simulink model "Model_vs_Real_control"  (R2019b)
settings: Solver=FixedStepAuto  StartTime=0.0  StopTime=10  FixedStep=1e-3  RelTol=1e-3
values from neighbouring files (symbols this model uses):
  N = 1/Tf    [HorizontalBeamControl.m]
  V_max = 10    [HorizontalBeamControl.m]
undefined symbols (not defined in the file or in its folder): Kd, Ki, Kp, Parameters, tf2_1, tf2_2
libraries: simulink x4
settings Model: Creator=Guido  LastModifiedBy=pietr

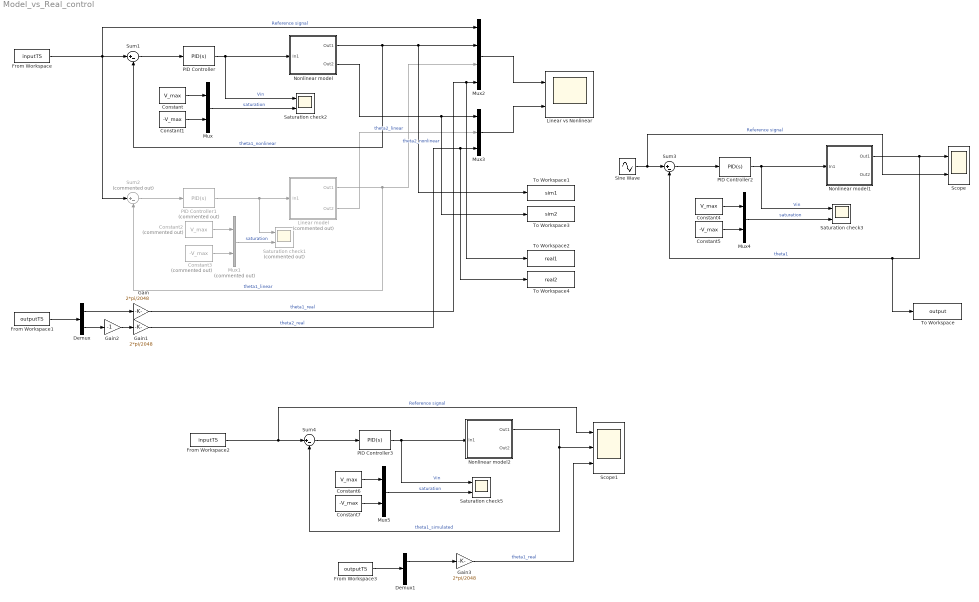
== system Model_vs_Real_control ==
  Constant : Constant  Value=V_max
  Constant1 : Constant  Value=-V_max
  Constant2 : Constant  Commented=on  Value=V_max
  Constant3 : Constant  Commented=on  Value=-V_max
  Constant4 : Constant  Value=V_max
  Constant5 : Constant  Value=-V_max
  Constant6 : Constant  Value=V_max
  Constant7 : Constant  Value=-V_max
  Demux : Demux  Outputs=2
  Demux1 : Demux  Outputs=2
  From Workspace : FromWorkspace  VariableName=inputTS  SampleTime=0
  From Workspace1 : FromWorkspace  VariableName=outputTS  SampleTime=0
  From Workspace2 : FromWorkspace  VariableName=inputTS  SampleTime=0
  From Workspace3 : FromWorkspace  VariableName=outputTS  SampleTime=0
  Gain : Gain  Gain=2*pi/2048
  Gain1 : Gain  Gain=2*pi/2048
  Gain2 : Gain  Gain=-1
  Gain3 : Gain  Gain=2*pi/2048
  Linear model : Subsystem  Commented=on
  Linear vs Nonlinear : Scope  NumInputPorts=2
  Mux : Mux  Inputs=2
  Mux1 : Mux  Commented=on  Inputs=2
  Mux2 : Mux
  Mux3 : Mux  Inputs=3
  Mux4 : Mux  Inputs=2
  Mux5 : Mux  Inputs=2
  Nonlinear model : Subsystem
  Nonlinear model1 : Subsystem
  Nonlinear model2 : Subsystem
  PID Controller : simulink/Continuous/PID Controller  Controller=PID  Form=Parallel  TimeDomain=Continuous-time  SampleTime=-1  IntegratorMethod=Forward Euler  FilterMethod=Forward Euler  ControllerParametersSource=internal  P=Kp  I=Ki  D=Kd  UseFilter=on  N=N  TunerSelectOption=Transfer Function Based (PID Tuner App)  InitialConditionSource=internal  InitialConditionForIntegrator=0  InitialConditionForFilter=0  DifferentiatorICPrevScaledInput=0  ExternalReset=none  TrackingMode=off  Kt=1  LimitOutput=on  UpperSaturationLimit=V_max  LowerSaturationLimit=-V_max  LinearizeAsGain=on  AntiWindupMode=back-calculation  Kb=1  POutMin=[]  POutMax=[]  IOutMin=[]  IOutMax=[]  DOutMin=[]  DOutMax=[]  NOutMin=[]  NOutMax=[]  SumOutMin=[]  SumOutMax=[]  SaturationOutMin=[]  SaturationOutMax=[]  PParamMin=[]  PParamMax=[]  IParamMin=[]  IParamMax=[]  DParamMin=[]  DParamMax=[]  NParamMin=[]  NParamMax=[]  KbParamMin=[]  KbParamMax=[]  KtParamMin=[]  KtParamMax=[]  KbOutMin=[]  KbOutMax=[]  KtOutMin=[]  KtOutMax=[]  IntegratorOutMin=[]  IntegratorOutMax=[]  FilterOutMin=[]  FilterOutMax=[]  SumI1OutMin=[]  SumI1OutMax=[]  SumI2OutMin=[]  SumI2OutMax=[]  SumI3OutMin=[]  SumI3OutMax=[]  SumI4OutMin=[]  SumI4OutMax=[]  SumDOutMin=[]  SumDOutMax=[]  DifferentiatorOutMin=[]  DifferentiatorOutMax=[]  FilterDiffOutCoefMin=[]  FilterDiffOutCoefMax=[]  ReciprocalOutMin=[]  ReciprocalOutMax=[]  SumDenOutMin=[]  SumDenOutMax=[]  SumNumOutMin=[]  SumNumOutMax=[]  DivideOutMin=[]  DivideOutMax=[]  IntegratorContinuousStateAttributes=''  IntegratorStateMustResolveToSignalObject=off  IntegratorRTWStateStorageClass=Auto  FilterContinuousStateAttributes=''  FilterStateMustResolveToSignalObject=off  FilterRTWStateStorageClass=Auto  ParallelPVariant=InternalParameters  IdealPVariant=Disabled  IVariant=InternalParameters  DVariant=InternalParameters  IntegratorVariant=Continuous  SatVariant=Enabled  AWVariant=BackCalculation  PCopyVariant=Disabled  TRVariant=Disabled  FdbkBlocksVariant=Forward  IdealPFdbkVariant=Disabled  SatFdbkVariant=Disabled  DerivativeFilterVariant=ContFilter  NVariant=InternalParameters  NCopyVariant=Disabled  FilterICVariant=InternalICsFilter  IntegratorICVariant=InternalICs  ExternalResetVariant=Disabled  TRSumVariant=Passthrough  SumFdbkVariant=Disabled  SumVariant=Sum_PID
  PID Controller1 : simulink/Continuous/PID Controller  Commented=on  Controller=PID  Form=Parallel  TimeDomain=Continuous-time  SampleTime=-1  IntegratorMethod=Forward Euler  FilterMethod=Forward Euler  ControllerParametersSource=internal  P=Kp  I=Ki  D=Kd  UseFilter=on  N=N  TunerSelectOption=Transfer Function Based (PID Tuner App)  InitialConditionSource=internal  InitialConditionForIntegrator=0  InitialConditionForFilter=0  DifferentiatorICPrevScaledInput=0  ExternalReset=none  TrackingMode=off  Kt=1  LimitOutput=on  UpperSaturationLimit=V_max  LowerSaturationLimit=-V_max  LinearizeAsGain=on  AntiWindupMode=back-calculation  Kb=1  POutMin=[]  POutMax=[]  IOutMin=[]  IOutMax=[]  DOutMin=[]  DOutMax=[]  NOutMin=[]  NOutMax=[]  SumOutMin=[]  SumOutMax=[]  SaturationOutMin=[]  SaturationOutMax=[]  PParamMin=[]  PParamMax=[]  IParamMin=[]  IParamMax=[]  DParamMin=[]  DParamMax=[]  NParamMin=[]  NParamMax=[]  KbParamMin=[]  KbParamMax=[]  KtParamMin=[]  KtParamMax=[]  KbOutMin=[]  KbOutMax=[]  KtOutMin=[]  KtOutMax=[]  IntegratorOutMin=[]  IntegratorOutMax=[]  FilterOutMin=[]  FilterOutMax=[]  SumI1OutMin=[]  SumI1OutMax=[]  SumI2OutMin=[]  SumI2OutMax=[]  SumI3OutMin=[]  SumI3OutMax=[]  SumI4OutMin=[]  SumI4OutMax=[]  SumDOutMin=[]  SumDOutMax=[]  DifferentiatorOutMin=[]  DifferentiatorOutMax=[]  FilterDiffOutCoefMin=[]  FilterDiffOutCoefMax=[]  ReciprocalOutMin=[]  ReciprocalOutMax=[]  SumDenOutMin=[]  SumDenOutMax=[]  SumNumOutMin=[]  SumNumOutMax=[]  DivideOutMin=[]  DivideOutMax=[]  IntegratorContinuousStateAttributes=''  IntegratorStateMustResolveToSignalObject=off  IntegratorRTWStateStorageClass=Auto  FilterContinuousStateAttributes=''  FilterStateMustResolveToSignalObject=off  FilterRTWStateStorageClass=Auto  ParallelPVariant=InternalParameters  IdealPVariant=Disabled  IVariant=InternalParameters  DVariant=InternalParameters  IntegratorVariant=Continuous  SatVariant=Enabled  AWVariant=BackCalculation  PCopyVariant=Disabled  TRVariant=Disabled  FdbkBlocksVariant=Forward  IdealPFdbkVariant=Disabled  SatFdbkVariant=Disabled  DerivativeFilterVariant=ContFilter  NVariant=InternalParameters  NCopyVariant=Disabled  FilterICVariant=InternalICsFilter  IntegratorICVariant=InternalICs  ExternalResetVariant=Disabled  TRSumVariant=Passthrough  SumFdbkVariant=Disabled  SumVariant=Sum_PID
  PID Controller2 : simulink/Continuous/PID Controller  Controller=PID  Form=Parallel  TimeDomain=Continuous-time  SampleTime=-1  IntegratorMethod=Forward Euler  FilterMethod=Forward Euler  ControllerParametersSource=internal  P=Kp  I=Ki  D=Kd  UseFilter=on  N=N  TunerSelectOption=Transfer Function Based (PID Tuner App)  InitialConditionSource=internal  InitialConditionForIntegrator=0  InitialConditionForFilter=0  DifferentiatorICPrevScaledInput=0  ExternalReset=none  TrackingMode=off  Kt=1  LimitOutput=on  UpperSaturationLimit=V_max  LowerSaturationLimit=-V_max  LinearizeAsGain=on  AntiWindupMode=back-calculation  Kb=1  POutMin=[]  POutMax=[]  IOutMin=[]  IOutMax=[]  DOutMin=[]  DOutMax=[]  NOutMin=[]  NOutMax=[]  SumOutMin=[]  SumOutMax=[]  SaturationOutMin=[]  SaturationOutMax=[]  PParamMin=[]  PParamMax=[]  IParamMin=[]  IParamMax=[]  DParamMin=[]  DParamMax=[]  NParamMin=[]  NParamMax=[]  KbParamMin=[]  KbParamMax=[]  KtParamMin=[]  KtParamMax=[]  KbOutMin=[]  KbOutMax=[]  KtOutMin=[]  KtOutMax=[]  IntegratorOutMin=[]  IntegratorOutMax=[]  FilterOutMin=[]  FilterOutMax=[]  SumI1OutMin=[]  SumI1OutMax=[]  SumI2OutMin=[]  SumI2OutMax=[]  SumI3OutMin=[]  SumI3OutMax=[]  SumI4OutMin=[]  SumI4OutMax=[]  SumDOutMin=[]  SumDOutMax=[]  DifferentiatorOutMin=[]  DifferentiatorOutMax=[]  FilterDiffOutCoefMin=[]  FilterDiffOutCoefMax=[]  ReciprocalOutMin=[]  ReciprocalOutMax=[]  SumDenOutMin=[]  SumDenOutMax=[]  SumNumOutMin=[]  SumNumOutMax=[]  DivideOutMin=[]  DivideOutMax=[]  IntegratorContinuousStateAttributes=''  IntegratorStateMustResolveToSignalObject=off  IntegratorRTWStateStorageClass=Auto  FilterContinuousStateAttributes=''  FilterStateMustResolveToSignalObject=off  FilterRTWStateStorageClass=Auto  ParallelPVariant=InternalParameters  IdealPVariant=Disabled  IVariant=InternalParameters  DVariant=InternalParameters  IntegratorVariant=Continuous  SatVariant=Enabled  AWVariant=BackCalculation  PCopyVariant=Disabled  TRVariant=Disabled  FdbkBlocksVariant=Forward  IdealPFdbkVariant=Disabled  SatFdbkVariant=Disabled  DerivativeFilterVariant=ContFilter  NVariant=InternalParameters  NCopyVariant=Disabled  FilterICVariant=InternalICsFilter  IntegratorICVariant=InternalICs  ExternalResetVariant=Disabled  TRSumVariant=Passthrough  SumFdbkVariant=Disabled  SumVariant=Sum_PID
  PID Controller3 : simulink/Continuous/PID Controller  Controller=PID  Form=Parallel  TimeDomain=Continuous-time  SampleTime=-1  IntegratorMethod=Forward Euler  FilterMethod=Forward Euler  ControllerParametersSource=internal  P=Kp  I=Ki  D=Kd  UseFilter=on  N=N  TunerSelectOption=Transfer Function Based (PID Tuner App)  InitialConditionSource=internal  InitialConditionForIntegrator=0  InitialConditionForFilter=0  DifferentiatorICPrevScaledInput=0  ExternalReset=none  TrackingMode=off  Kt=1  LimitOutput=on  UpperSaturationLimit=V_max  LowerSaturationLimit=-V_max  LinearizeAsGain=on  AntiWindupMode=back-calculation  Kb=1  POutMin=[]  POutMax=[]  IOutMin=[]  IOutMax=[]  DOutMin=[]  DOutMax=[]  NOutMin=[]  NOutMax=[]  SumOutMin=[]  SumOutMax=[]  SaturationOutMin=[]  SaturationOutMax=[]  PParamMin=[]  PParamMax=[]  IParamMin=[]  IParamMax=[]  DParamMin=[]  DParamMax=[]  NParamMin=[]  NParamMax=[]  KbParamMin=[]  KbParamMax=[]  KtParamMin=[]  KtParamMax=[]  KbOutMin=[]  KbOutMax=[]  KtOutMin=[]  KtOutMax=[]  IntegratorOutMin=[]  IntegratorOutMax=[]  FilterOutMin=[]  FilterOutMax=[]  SumI1OutMin=[]  SumI1OutMax=[]  SumI2OutMin=[]  SumI2OutMax=[]  SumI3OutMin=[]  SumI3OutMax=[]  SumI4OutMin=[]  SumI4OutMax=[]  SumDOutMin=[]  SumDOutMax=[]  DifferentiatorOutMin=[]  DifferentiatorOutMax=[]  FilterDiffOutCoefMin=[]  FilterDiffOutCoefMax=[]  ReciprocalOutMin=[]  ReciprocalOutMax=[]  SumDenOutMin=[]  SumDenOutMax=[]  SumNumOutMin=[]  SumNumOutMax=[]  DivideOutMin=[]  DivideOutMax=[]  IntegratorContinuousStateAttributes=''  IntegratorStateMustResolveToSignalObject=off  IntegratorRTWStateStorageClass=Auto  FilterContinuousStateAttributes=''  FilterStateMustResolveToSignalObject=off  FilterRTWStateStorageClass=Auto  ParallelPVariant=InternalParameters  IdealPVariant=Disabled  IVariant=InternalParameters  DVariant=InternalParameters  IntegratorVariant=Continuous  SatVariant=Enabled  AWVariant=BackCalculation  PCopyVariant=Disabled  TRVariant=Disabled  FdbkBlocksVariant=Forward  IdealPFdbkVariant=Disabled  SatFdbkVariant=Disabled  DerivativeFilterVariant=ContFilter  NVariant=InternalParameters  NCopyVariant=Disabled  FilterICVariant=InternalICsFilter  IntegratorICVariant=InternalICs  ExternalResetVariant=Disabled  TRSumVariant=Passthrough  SumFdbkVariant=Disabled  SumVariant=Sum_PID
  Saturation check1 : Scope  Commented=on  NumInputPorts=2
  Saturation check2 : Scope  NumInputPorts=2
  Saturation check3 : Scope  NumInputPorts=2
  Saturation check5 : Scope  NumInputPorts=2
  Scope : Scope  NumInputPorts=2
  Scope1 : Scope  NumInputPorts=3
  Sine Wave : Sin  Frequency=4  SampleTime=0
  Sum1 : Sum  Inputs=|+-
  Sum2 : Sum  Commented=on  Inputs=|+-
  Sum3 : Sum  Inputs=|+-
  Sum4 : Sum  Inputs=|+-
  To Workspace : ToWorkspace  VariableName=output  SampleTime=0.02
      settings: Save2DSignal=2-D array (concatenate along first dimension)
  To Workspace1 : ToWorkspace  VariableName=sim1  SampleTime=-1
      settings: Save2DSignal=2-D array (concatenate along first dimension)
  To Workspace2 : ToWorkspace  VariableName=real1  SampleTime=-1
      settings: Save2DSignal=2-D array (concatenate along first dimension)
  To Workspace3 : ToWorkspace  VariableName=sim2  SampleTime=-1
      settings: Save2DSignal=2-D array (concatenate along first dimension)
  To Workspace4 : ToWorkspace  VariableName=real2  SampleTime=-1
      settings: Save2DSignal=2-D array (concatenate along first dimension)
  wires:
  Mux3/1 -> Linear vs Nonlinear/2
  From Workspace/1 -> Sum2/1, Mux2/1, Sum1/1  "Reference signal"
  Mux1/1 -> Saturation check1/2  "saturation"
  Linear model/1(Out1) -> Sum2/2, Mux2/3  "theta1_linear"
  Sum1/1 -> PID Controller/1
  Mux2/1 -> Linear vs Nonlinear/1
  Sum2/1 -> PID Controller1/1
  Constant2/1 -> Mux1/1
  Constant3/1 -> Mux1/2
  Linear model/2(Out2) -> Mux3/2  "theta2_linear"
  Nonlinear model/1(Out1) -> Sum1/2, To Workspace1/1, Mux2/2  "theta1_nonlinear"
  Mux/1 -> Saturation check2/2  "saturation"
  Nonlinear model/2(Out2) -> To Workspace3/1, Mux3/1  "theta2_nonlinear"
  Constant1/1 -> Mux/2
  Constant/1 -> Mux/1
  From Workspace1/1 -> Demux/1
  Demux/1 -> Gain/1
  Demux/2 -> Gain2/1
  Gain/1 -> To Workspace2/1, Mux2/4  "theta1_real"
  Gain1/1 -> To Workspace4/1, Mux3/3  "theta2_real"
  Gain2/1 -> Gain1/1
  PID Controller/1 -> Saturation check2/1, Nonlinear model/1(In1)  "Vin"
  PID Controller1/1 -> Linear model/1(In1), Saturation check1/1
  Sine Wave/1 -> Scope/2, Sum3/1  "Reference signal"
  Nonlinear model1/1(Out1) -> Scope/1, To Workspace/1, Sum3/2  "theta1"
  Constant4/1 -> Mux4/1
  Mux4/1 -> Saturation check3/2  "saturation"
  PID Controller2/1 -> Saturation check3/1, Nonlinear model1/1(In1)  "Vin"
  Sum3/1 -> PID Controller2/1
  Constant5/1 -> Mux4/2
  PID Controller3/1 -> Saturation check5/1, Nonlinear model2/1(In1)  "Vin"
  From Workspace3/1 -> Demux1/1
  Demux1/1 -> Gain3/1
  Gain3/1 -> Scope1/3  "theta1_real"
  Mux5/1 -> Saturation check5/2  "saturation"
  Sum4/1 -> PID Controller3/1
  Nonlinear model2/1(Out1) -> Sum4/2, Scope1/2  "theta1_simulated"
  Constant7/1 -> Mux5/2
  From Workspace2/1 -> Scope1/1, Sum4/1  "Reference signal"
  Constant6/1 -> Mux5/1

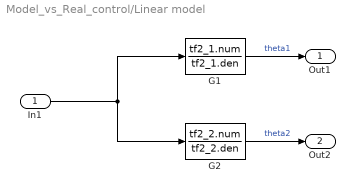
== system Model_vs_Real_control/Linear model ==
  In1 : Inport
  G1 : TransferFcn  Numerator=tf2_1.num  Denominator=tf2_1.den
  G2 : TransferFcn  Numerator=tf2_2.num  Denominator=tf2_2.den
  Out1 : Outport
  Out2 : Outport  Port=2
  wires:
  In1/1 -> G2/1, G1/1
  G1/1 -> Out1/1  "theta1"
  G2/1 -> Out2/1  "theta2"

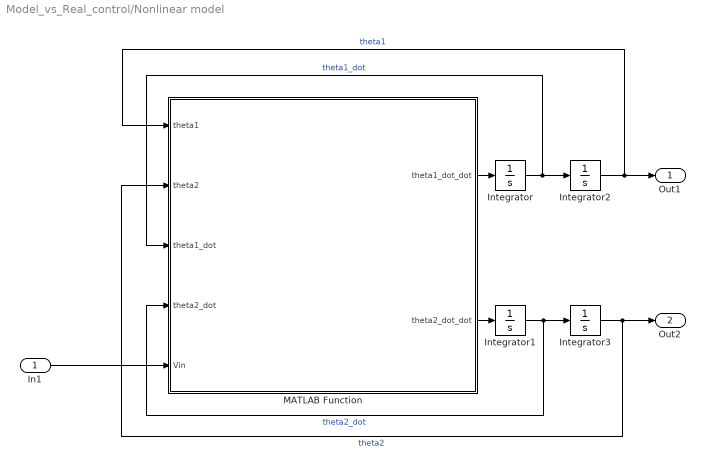
== system Model_vs_Real_control/Nonlinear model ==
  In1 : Inport
  Integrator{,1..3} (4 alike) : Integrator
  MATLAB Function : MATLAB Function  TreatAsAtomicUnit=on  mask{Pars=Parameters}
      mask prompts: Pars "Struct containing model parameters"
  Out1 : Outport
  Out2 : Outport  Port=2
  wires:
  Integrator/1 -> MATLAB Function/3(theta1_dot), Integrator2/1  "theta1_dot"
  Integrator1/1 -> MATLAB Function/4(theta2_dot), Integrator3/1  "theta2_dot"
  MATLAB Function/1(theta1_dot_dot) -> Integrator/1
  Integrator3/1 -> Out2/1, MATLAB Function/2(theta2)  "theta2"
  MATLAB Function/2(theta2_dot_dot) -> Integrator1/1
  Integrator2/1 -> MATLAB Function/1(theta1), Out1/1  "theta1"
  In1/1 -> MATLAB Function/5(Vin)

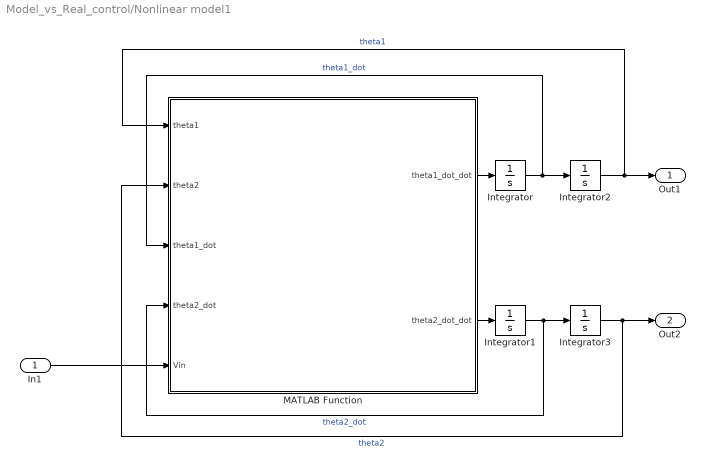
== system Model_vs_Real_control/Nonlinear model1 ==
  In1 : Inport
  Integrator{,1..3} (4 alike) : Integrator
  MATLAB Function : MATLAB Function  TreatAsAtomicUnit=on  mask{Pars=Parameters}
      mask prompts: Pars "Struct containing model parameters"
  Out1 : Outport
  Out2 : Outport  Port=2
  wires:
  Integrator/1 -> MATLAB Function/3(theta1_dot), Integrator2/1  "theta1_dot"
  Integrator1/1 -> MATLAB Function/4(theta2_dot), Integrator3/1  "theta2_dot"
  MATLAB Function/1(theta1_dot_dot) -> Integrator/1
  Integrator3/1 -> Out2/1, MATLAB Function/2(theta2)  "theta2"
  MATLAB Function/2(theta2_dot_dot) -> Integrator1/1
  Integrator2/1 -> MATLAB Function/1(theta1), Out1/1  "theta1"
  In1/1 -> MATLAB Function/5(Vin)

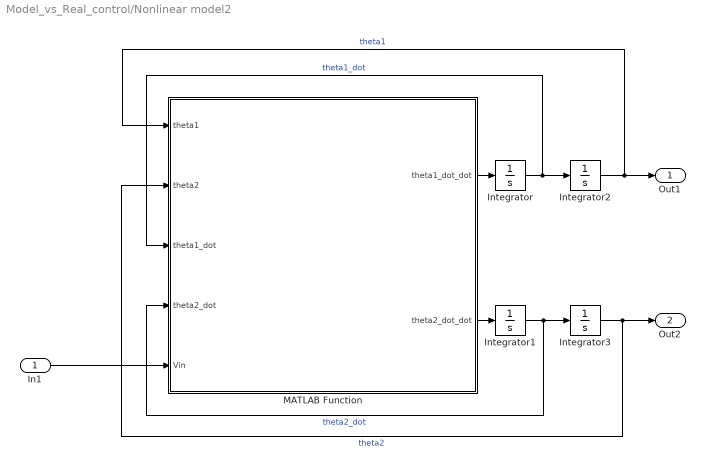
== system Model_vs_Real_control/Nonlinear model2 ==
  In1 : Inport
  Integrator{,1..3} (4 alike) : Integrator
  MATLAB Function : MATLAB Function  TreatAsAtomicUnit=on  mask{Pars=Parameters}
      mask prompts: Pars "Struct containing model parameters"
  Out1 : Outport
  Out2 : Outport  Port=2
  wires:
  Integrator/1 -> MATLAB Function/3(theta1_dot), Integrator2/1  "theta1_dot"
  Integrator1/1 -> MATLAB Function/4(theta2_dot), Integrator3/1  "theta2_dot"
  MATLAB Function/1(theta1_dot_dot) -> Integrator/1
  Integrator3/1 -> Out2/1, MATLAB Function/2(theta2)  "theta2"
  MATLAB Function/2(theta2_dot_dot) -> Integrator1/1
  Integrator2/1 -> MATLAB Function/1(theta1), Out1/1  "theta1"
  In1/1 -> MATLAB Function/5(Vin)

== matlab function Model_vs_Real_control/Nonlinear model1/MATLAB Function ==
  data: theta1 input; theta1_dot_dot output; theta2 input; theta1_dot input; theta2_dot input; Vin input; theta2_dot_dot output; Pars parameter
function [theta1_dot_dot,theta2_dot_dot] = fcn(theta1, theta2, theta1_dot, theta2_dot,Vin, Pars)

   k1 = Pars.Jeq + Pars.m2*(Pars.l1^2 + Pars.x2^2*sin(theta2)^2);
   k2 = Pars.m2*Pars.l1*Pars.x2*cos(theta2);
   k3 = 2*Pars.m2*Pars.x2^2*sin(theta2)*cos(theta2)*theta1_dot*theta2_dot - Pars.m2*Pars.l1*Pars.x2*sin(theta2)*theta2_dot^2 +Pars.Ks*theta1 - Pars.Km/Pars.Rm*Vin + (Pars.Km^2)/Pars.Rm*theta1_dot + Pars.Kf1*theta1_dot;
   k4 = Pars.m2*Pars.l1*Pars.x2*cos(theta2);
   k5 = Pars.m2*Pars.x2^2 + Pars.I2;
   k6 = - Pars.m2*Pars.x2^2*sin(theta2)*cos(theta2)*theta1_dot^2 + Pars.m2*Pars.g*Pars.x2*sin(theta2) + Pars.Kf2*theta2_dot;


theta1_dot_dot = (k2*k6 - k3*k5)/(k1*k5 - k2*k4);
theta2_dot_dot = -(k1*k6 - k3*k4)/(k1*k5 - k2*k4);

== matlab function Model_vs_Real_control/Nonlinear model/MATLAB Function ==
  data: theta1 input; theta1_dot_dot output; theta2 input; theta1_dot input; theta2_dot input; Vin input; theta2_dot_dot output; Pars parameter
function [theta1_dot_dot,theta2_dot_dot] = fcn(theta1, theta2, theta1_dot, theta2_dot,Vin, Pars)

   k1 = Pars.Jeq + Pars.m2*(Pars.l1^2 + Pars.x2^2*sin(theta2)^2);
   k2 = Pars.m2*Pars.l1*Pars.x2*cos(theta2);
   k3 = 2*Pars.m2*Pars.x2^2*sin(theta2)*cos(theta2)*theta1_dot*theta2_dot - Pars.m2*Pars.l1*Pars.x2*sin(theta2)*theta2_dot^2 +Pars.Ks*theta1 - Pars.Km/Pars.Rm*Vin + (Pars.Km^2)/Pars.Rm*theta1_dot + Pars.Kf1*theta1_dot;
   k4 = Pars.m2*Pars.l1*Pars.x2*cos(theta2);
   k5 = Pars.m2*Pars.x2^2 + Pars.I2;
   k6 = - Pars.m2*Pars.x2^2*sin(theta2)*cos(theta2)*theta1_dot^2 + Pars.m2*Pars.g*Pars.x2*sin(theta2) + Pars.Kf2*theta2_dot;


theta1_dot_dot = (k2*k6 - k3*k5)/(k1*k5 - k2*k4);
theta2_dot_dot = -(k1*k6 - k3*k4)/(k1*k5 - k2*k4);

== matlab function Model_vs_Real_control/Nonlinear model2/MATLAB Function ==
  data: theta1 input; theta1_dot_dot output; theta2 input; theta1_dot input; theta2_dot input; Vin input; theta2_dot_dot output; Pars parameter
function [theta1_dot_dot,theta2_dot_dot] = fcn(theta1, theta2, theta1_dot, theta2_dot,Vin, Pars)

   k1 = Pars.Jeq + Pars.m2*(Pars.l1^2 + Pars.x2^2*sin(theta2)^2);
   k2 = Pars.m2*Pars.l1*Pars.x2*cos(theta2);
   k3 = 2*Pars.m2*Pars.x2^2*sin(theta2)*cos(theta2)*theta1_dot*theta2_dot - Pars.m2*Pars.l1*Pars.x2*sin(theta2)*theta2_dot^2 +Pars.Ks*theta1 - Pars.Km/Pars.Rm*Vin + (Pars.Km^2)/Pars.Rm*theta1_dot + Pars.Kf1*theta1_dot;
   k4 = Pars.m2*Pars.l1*Pars.x2*cos(theta2);
   k5 = Pars.m2*Pars.x2^2 + Pars.I2;
   k6 = - Pars.m2*Pars.x2^2*sin(theta2)*cos(theta2)*theta1_dot^2 + Pars.m2*Pars.g*Pars.x2*sin(theta2) + Pars.Kf2*theta2_dot;


theta1_dot_dot = (k2*k6 - k3*k5)/(k1*k5 - k2*k4);
theta2_dot_dot = -(k1*k6 - k3*k4)/(k1*k5 - k2*k4);
